simulink model "pt1_discrete_tustin"  (R2019a)
settings: Solver=FixedStepDiscrete  StartTime=0.0  StopTime=10e-3  FixedStep=P_Ta  RelTol=1e-3  EnableMultiTasking=on
InitFcn:
  | pt1_data;
values from neighbouring files (symbols this model uses):
  P_k = 1    [pt1_data.m]
  P_T = 100e-6    (= 0.0001)    [pt1_data.m]
  P_Ta = 5e-6    (= 5e-06)    [pt1_data.m]
settings Model: Creator=ftraenkle  LastModifiedBy=ftraenkle
settings DataIOCC: LimitDataPoints=on  SaveFormat=Array  InspectSignalLogs=on  ReturnWorkspaceOutputs=off
settings OptimizationCC: LifeSpan=inf
settings DebuggingCC: UnderspecifiedInitializationDetection=Classic  MergeDetectMultiDrivingBlocksExec=none  SolverPrmCheckMsg=warning  MultiTaskDSMMsg=warning  MultiTaskCondExecSysMsg=none  AllowSymbolicDim=off  StateNameClashWarn=warning  SFUnexpectedBacktrackingDiag=warning  SFNoUnconditionalDefaultTransitionDiag=warning  SFExecutionAtInitializationDiag=none  ArithmeticOperatorsInVariantConditions=warning
settings HardwareCC: ProdBitPerPointer=32  ProdBitPerSizeT=32  ProdBitPerPtrDiffT=32  ProdLargestAtomicFloat=None  ProdIntDivRoundTo=Undefined  ProdEndianess=Unspecified  ProdWordSize=32  ProdHWDeviceType=32-bit Generic
settings ModelReferenceCC: PropagateSignalLabelsOutOfModel=off
settings SFSimCC: SimUseLocalCustomCode=off
settings RTWCC: RTWUseLocalCustomCode=off
settings CodeAppCC: StateflowObjectComments=on
settings GRTTargetCC: TargetLangStandard=C89/C90 (ANSI)
settings ConfigComp: CovMetricSettings=dw  CovSaveCumulativeToWorkspaceVar=on  CovSaveSingleToWorkspaceVar=on  CovExternalEMLEnable=off

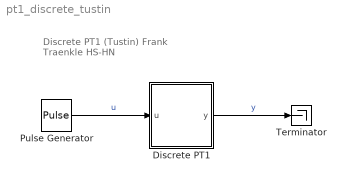
== system pt1_discrete_tustin ==
  note: Discrete PT1 (Tustin)
      | Frank Traenkle
      | HS-HN
  Discrete PT1 : Subsystem  TreatAsAtomicUnit=on  SystemSampleTime=P_Ta
  Pulse Generator : DiscretePulseGenerator  PulseType=Time based  Period=2e-3  PulseWidth=50
  Terminator : Terminator
  wires:
  Pulse Generator/1 -> Discrete PT1/1(u)  "u"
  Discrete PT1/1(y) -> Terminator/1  "y"

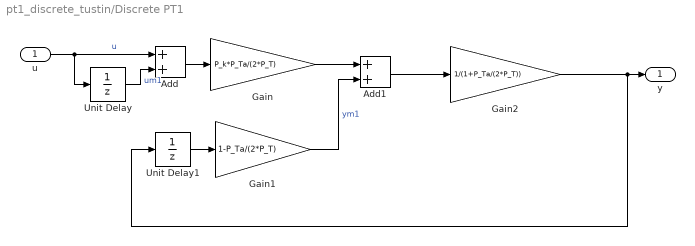
== system pt1_discrete_tustin/Discrete PT1 ==
  u : Inport
  Add : Sum
  Add1 : Sum
  Gain : Gain  Gain=P_k*P_Ta/(2*P_T)
  Gain1 : Gain  Gain=1-P_Ta/(2*P_T)
  Gain2 : Gain  Gain=1/(1+P_Ta/(2*P_T))
  Unit Delay : UnitDelay  SampleTime=-1  HasFrameUpgradeWarning=on
  Unit Delay1 : UnitDelay  SampleTime=-1  HasFrameUpgradeWarning=on
  y : Outport
  wires:
  u/1 -> Add/1, Unit Delay/1  "u"
  Unit Delay/1 -> Add/2  "um1"
  Add/1 -> Gain/1
  Gain/1 -> Add1/1
  Gain2/1 -> Unit Delay1/1, y/1
  Add1/1 -> Gain2/1
  Unit Delay1/1 -> Gain1/1
  Gain1/1 -> Add1/2  "ym1"
